simulink model "IEEE9_16b_0"  (R2020a)
settings: Solver=ode15s  StartTime=0.0  StopTime=5  MaxStep=1e-4  RelTol=1e-3
libraries: powerlib x23, sps_avr x3, simulink_extras x2, powerlib_meascontrol x2
settings Model: Creator=Pankaj  LastModifiedBy=ahmed
settings DataIOCC: ReturnWorkspaceOutputs=off
settings DebuggingCC: UnconnectedInputMsg=none  UnconnectedOutputMsg=none  UnconnectedLineMsg=none  ArithmeticOperatorsInVariantConditions=warning
settings SFSimCC: SimUseLocalCustomCode=off  CustomCodeUndefinedFunction=UseInterfaceOnly
settings RTWCC: RTWUseLocalCustomCode=off
settings CodeAppCC: StateflowObjectComments=on
settings SimscapeCC: SimscapeNormalizeSystem=off

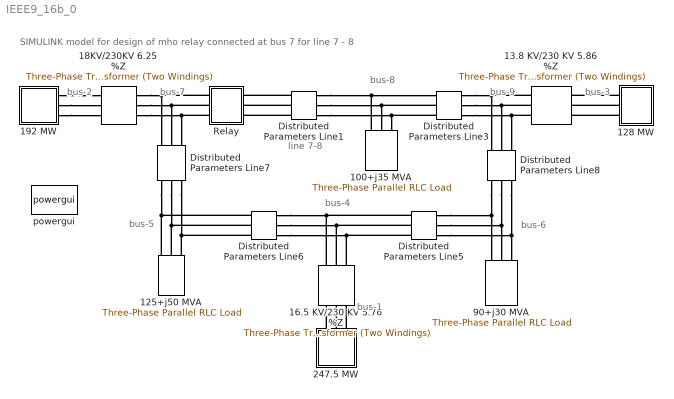
== system IEEE9_16b_0 ==
  note: SIMULINK model for design of mho relay connected at bus 7 for line 7 - 8
  note: bus-2
  note: bus-7
  note: bus-8
  note: bus-9
  note: bus-1
  note: bus-3
  note: bus-4
  note: bus-6
  note: bus-5
  note: line 7-8
  100+j35 MVA : powerlib/Elements/Three-Phase Parallel RLC Load  LConnTagsString=A|B|C  Configuration=Y (grounded)  NominalVoltage=(230000)*0.993698  Vabc=[1e3 1e3 1e3]  Vabcp=[1e3 1e3 1e3]  NominalFrequency=60  UnbalancedPower=off  ActivePower=100e6  InductivePower=35e6  CapacitivePower=0  Pabc=[10e3 9e3 11e3]  QLabc=[100 90 110]  QCabc=[100 90 110]  Pabcp=[10e3 9e3 11e3]  QLabcp=[100 90 110]  QCabcp=[100 90 110]  Measurements=None  LoadType=constant PQ
  125+j50 MVA : powerlib/Elements/Three-Phase Parallel RLC Load  LConnTagsString=A|B|C  Configuration=Y (grounded)  NominalVoltage=(223027)*1  Vabc=[1e3 1e3 1e3]  Vabcp=[1e3 1e3 1e3]  NominalFrequency=60  UnbalancedPower=off  ActivePower=125e6  InductivePower=50e6  CapacitivePower=0  Pabc=[10e3 9e3 11e3]  QLabc=[100 90 110]  QCabc=[100 90 110]  Pabcp=[10e3 9e3 11e3]  QLabcp=[100 90 110]  QCabcp=[100 90 110]  Measurements=None  LoadType=constant PQ
  128 MW : Subsystem
  13.8 KV/230 KV 5.86 %Z : powerlib/Elements/Three-Phase Transformer (Two Windings)  Winding1Connection=Yg  Winding2Connection=Yg  CoreType=Three single-phase transformers  SetSaturation=off  Hysteresis=off  DataFile='hysteresis'  SetInitialFlux=off  Measurements=None  UNITS=pu  NominalPower=[ 100e6 , 60 ]  Winding1=[13.8e3 , 1e-6 , 0 ]  Winding2=[ 230e3 , 1e-6, 0.0586 ]  Rm=500  Lm=500  L0=0.5  Saturation=[ 0,0 ; 0.0024,1.2 ; 1.0,1.52 ]  InitialFluxes=[ 0.8 , -0.8 , 0.7 ]  BreakLoop=off  DiscreteSolver=Trapezoidal iterative  DataType=off  TransfoNumber=1
  "16.5 KV/230 KV 5.76 %Z     " : powerlib/Elements/Three-Phase Transformer (Two Windings)  Winding1Connection=Yg  Winding2Connection=Yg  CoreType=Three single-phase transformers  SetSaturation=off  Hysteresis=off  DataFile='hysteresis'  SetInitialFlux=off  Measurements=None  UNITS=pu  NominalPower=[ 100e6 , 60 ]  Winding1=[16.5e3 , 1e-6, 0 ]  Winding2=[ 230e3 ,1e-6, 0.0576 ]  Rm=500  Lm=500  L0=0.5  Saturation=[ 0,0 ; 0.0024,1.2 ; 1.0,1.52 ]  InitialFluxes=[ 0.8 , -0.8 , 0.7 ]  BreakLoop=off  DiscreteSolver=Trapezoidal iterative  DataType=off  TransfoNumber=1
  18KV/230KV 6.25 %Z : powerlib/Elements/Three-Phase Transformer (Two Windings)  Winding1Connection=Yg  Winding2Connection=Yg  CoreType=Three single-phase transformers  SetSaturation=off  Hysteresis=off  DataFile='hysteresis'  SetInitialFlux=off  Measurements=None  UNITS=pu  NominalPower=[ 100e6 , 60 ]  Winding1=[ 18e3 , 1e-6 , 0]  Winding2=[ 230e3 , 1e-6, 0.0625 ]  Rm=500  Lm=500  L0=0.5  Saturation=[ 0,0 ; 0.0024,1.2 ; 1.0,1.52 ]  InitialFluxes=[ 0.8 , -0.8 , 0.7 ]  BreakLoop=off  DiscreteSolver=Trapezoidal iterative  DataType=off  TransfoNumber=1
  192 MW : Subsystem
  247.5 MW : Subsystem
  90+j30 MVA : powerlib/Elements/Three-Phase Parallel RLC Load  LConnTagsString=A|B|C  Configuration=Y (grounded)  NominalVoltage=(226177)*0.999999  Vabc=[1e3 1e3 1e3]  Vabcp=[1e3 1e3 1e3]  NominalFrequency=60  UnbalancedPower=off  ActivePower=90e6  InductivePower=30e6  CapacitivePower=0  Pabc=[10e3 9e3 11e3]  QLabc=[100 90 110]  QCabc=[100 90 110]  Pabcp=[10e3 9e3 11e3]  QLabcp=[100 90 110]  QCabcp=[100 90 110]  Measurements=None  LoadType=constant PQ
  Distributed Parameters Line1 : powerlib/Elements/Distributed Parameters Line  Phases=3  Frequency=60  Resistance=[0.044965 0.11241]  Inductance="[1.01e-3  2.02e-3]"  Capacitance=[12.74e-9 7.751e-9]  Length=100  x1=[-0.0004 1.93656449270455e-06 23508.2160177902 -52538.75935175;-0.00035 1.67378461087068e-06 24494.3184666325 -52086.3350065214;-0.0003 1.4104100413345e-06 25471.7182007562 -51615.4046344802;-0.00025 1.14653435982647e-06 26440.0679546897 -51126.1355549453;-0.0002 8.82251320119748e-07 27399.0236783764 -50618.7016028908;-0.00015 6.17654820719931e-07 28348.2446594139 -50093.2830671837;-0.0001 3.52838871503349e-07 29287.3936441074 -49550.0666265279;-5e-05 8.78975603158065e-08 30216.1369572946 -48989.2452831382]  x2=[-0.0004 4.18624145948892e-06 28259.244689254 -52398.8670670216;-0.00035 3.9633430905482e-06 29241.8663646278 -51856.9185470287;-0.0003 3.73903656467934e-06 30214.0985441207 -51296.5455107989;-0.00025 3.51340157692291e-06 31175.595798269 -50717.9470562037;-0.0002 3.28651829431568e-06 32126.0165116764 -50121.3287565189;-0.00015 3.05846732740762e-06 33065.023004389 -49506.9025873855;-0.0001 2.82932970162139e-06 33992.2816518711 -48874.8868514958;-5e-05 2.59918682846436e-06 34907.4630035407 -48225.5061010312]  x3=[-0.0004 -1.73044531826081e-08 87.9731080176391 -312.019576771818;-0.00035 -1.71851910893741e-08 93.8385916181453 -310.305999768085;-0.0003 -1.70598231795753e-08 99.6707348138731 -308.482172520194;-0.00025 -1.69283939958332e-08 105.467465472116 -306.54874302528;-0.0002 -1.67909502343109e-08 111.226724042071 -304.506398221637;-0.00015 -1.66475407281225e-08 116.946464286594 -302.355863744649;-0.0001 -1.64982164299825e-08 122.624654009211 -300.097903668976;-5e-05 -1.63430303941032e-08 128.259275776149 -297.733320237081]  x4=[-0.0004 3.28235405138543e-08 68.6553647797155 -68.5872480221798;-0.00035 3.17845507984995e-08 69.935937439127 -67.2810236786274;-0.0003 3.07342681835919e-08 71.1916621929746 -65.9508947077285;-0.00025 2.96730658295436e-08 72.4220928882326 -64.5973336979729;-0.0002 2.86013207764978e-08 73.6267923587337 -63.2208215631423;-0.00015 2.75194138103686e-08 74.8053325804924 -61.8218473714436;-0.0001 2.64277293275496e-08 75.9572948237797 -60.400908171746;-5e-05 2.53266551983393e-08 77.0822698018957 -58.9585088169809]  x5=0.000395689524753941  V1=ones(3,3)  V2=ones(3,3)  I1=ones(3,3)  I2=ones(3,3)  nHarmo=1  Measurements=None
  Distributed Parameters Line3 : powerlib/Elements/Distributed Parameters Line  Phases=3  Frequency=60  Resistance=[ 0.062951 0.15737]  Inductance="[ 1.414e-3  3.53e-3]"  Capacitance=[12.74e-9 7.751e-9]  Length=100  x1=[-0.00055 -3.66870332071984e-11 0 0;-0.0005 -3.60227656771721e-11 0 0;-0.00045 -3.53456994300274e-11 0 0;-0.0004 -3.46560750241779e-11 0 0;-0.00035 -3.39541374798913e-11 0 0;-0.0003 -3.32401361922348e-11 0 0;-0.00025 -3.25143248424659e-11 0 0;-0.0002 -3.17769613079014e-11 0 0;-0.00015 -3.10283075702939e-11 0 0;-0.0001 -3.02686296227516e-11 0 0;-5e-05 -2.9498197375232e-11 0 0]  x2=[-0.00055 6.0309326536538e-11 0 0;-0.0005 6.04326397123915e-11 0 0;-0.00045 6.05344814591124e-11 26135.3734716676 3233.45213495311;-0.0004 6.06148155928129e-11 26069.7846141014 3725.4882649243;-0.00035 6.0673613571158e-11 25994.9332861961 4216.20074665431;-0.0003 6.07108545035057e-11 25910.8460822721 4705.41523233496;-0.00025 6.07265251583303e-11 25817.5528781127 5192.95790638897;-0.0002 6.07206199679226e-11 25715.0868203491 5678.65554722571;-0.00015 6.06931410303687e-11 25603.4843146836 6162.33558878611;-0.0001 6.06440981088042e-11 25482.785012955 6643.82618185451;-5e-05 6.05735086279458e-11 25353.0317990507 7122.95625511585]  x3=[-0.00055 1.99765696866532e-13 0 0;-0.0005 2.12696705234761e-13 0 0;-0.00045 2.255521434764e-13 116.024829696429 -474.092172875078;-0.0004 2.38327444115455e-13 124.940123526668 -471.821073684818;-0.00035 2.5101806814844e-13 133.811026725934 -469.38233871371;-0.0003 2.63619506657064e-13 142.634387504562 -466.776834432677;-0.00025 2.76127282410229e-13 151.407070964479 -464.005486564982;-0.0002 2.88536951454765e-13 160.125960213026 -461.069279757328;-0.00015 3.00844104694353e-13 168.787957470368 -457.969257230012;-0.0001 3.13044369456047e-13 177.389985170124 -454.706520406277;-5e-05 3.25133411043871e-13 185.928987052813 -451.28222852098]  x4=[-0.00055 -2.34485159346315e-13 0 0;-0.0005 -2.46871311009831e-13 0 0;-0.00045 -2.59169750472053e-13 -37.9101805249176 477.43059089476;-0.0004 -2.71376108155999e-13 -46.9022764073901 476.631236412791;-0.00035 -2.83486047200907e-13 -55.8777081343857 475.662537122061;-0.0003 -2.95495265003096e-13 -64.8332867777495 474.524837196814;-0.00025 -3.07399494744665e-13 -73.7658304630324 473.218540856417;-0.0002 -3.19194506909471e-13 -82.6721654999966 471.74411222174;-0.00015 -3.30876110785854e-13 -91.5491275102119 470.102075150256;-0.0001 -3.42440155955581e-13 -100.393562551345 468.293013049917;-5e-05 -3.53882533768465e-13 -109.202328237739 466.317568671875]  x5=0.000523077718890797  V1=ones(3,3)  V2=ones(3,3)  I1=ones(3,3)  I2=ones(3,3)  nHarmo=1  Measurements=None
  Distributed Parameters Line5 : powerlib/Elements/Distributed Parameters Line  Phases=3  Frequency=60  Resistance=[ 0.08993 0.224825]  Inductance="[ 1.29e-3  3.22e-3]"  Capacitance=[12.74e-9 7.751e-9]  Length=100  x1=[-0.0005 9.3934579093273e-11 48708.3011698947 -2975.91430508471;-0.00045 9.415092660108e-11 48755.7392345492 -2057.30749504863;-0.0004 9.43338227329765e-11 48785.85461721 -1137.96973345567;-0.00035 9.44832025068375e-11 48798.6366180249 -218.227656634997;-0.0003 9.45990128487408e-11 48794.0806956099 701.591955432963;-0.00025 9.46812126118233e-11 48772.1884686624 1621.16229521987;-0.0002 9.47297725909006e-11 48732.9677153866 2540.15664376264;-0.00015 9.47446755328433e-11 48676.4323707293 3458.24848674514;-0.0001 9.47259161427072e-11 48602.6025214293 4375.11163050716;-5e-05 9.46735010856142e-11 48511.5043988804 5290.42031793947]  x2=[-0.0005 5.85167207852729e-11 40015.4206134486 -3326.82844604819;-0.00045 5.87167241813035e-11 40071.0170008075 -2572.00768036554;-0.0004 5.8895865804819e-11 40112.3763466289 -1816.27309260098;-0.00035 5.90540820076537e-11 40139.4839561341 -1059.89319165501;-0.0003 5.9191316576344e-11 40152.3301981187 -303.136715704854;-0.00025 5.93075207521012e-11 40150.9105083739 453.727463276971;-0.0002 5.9402653248135e-11 40135.2253913087 1210.43043505157;-0.00015 5.94766802643224e-11 40105.2804197707 1966.7033466562;-0.0001 5.95295754992172e-11 40061.0862330655 2722.27749792646;-5e-05 5.95613201593942e-11 40002.6585331773 3476.88443696415]  x3=[-0.0005 8.69475041814123e-14 110.762184106389 149.128598468394;-0.00045 8.25552456581707e-14 107.931686449283 151.189801864665;-0.0004 7.81336556492433e-14 105.062841177911 153.197288244241;-0.00035 7.36843051245063e-14 102.156667579338 155.150344356771;-0.0003 6.92087749170151e-14 99.2141982032043 157.048276290718;-0.00025 6.47086551613417e-14 96.2364784948694 158.890409719903;-0.0002 6.01855447286073e-14 93.2245664239666 160.676090143089;-0.00015 5.56410506584114e-14 90.1795321085132 162.404683116526;-0.0001 5.1076787587858e-14 87.1024574347021 164.075574479361;-5e-05 4.64943771778828e-14 83.9944356725131 165.688170571848]  x4=[-0.0005 1.05776183792212e-13 160.713797226438 -189.568367256825;-0.00045 1.09353327185716e-13 164.258290736407 -186.505475277131;-0.0004 1.1289161786277e-13 167.744424057812 -183.37631879014;-0.00035 1.16389798685544e-13 171.170958584084 -180.18200957025;-0.0003 1.19846626767049e-13 174.536676883822 -176.923682540318;-0.00025 1.23260873912727e-13 177.84038313334 -173.602495368422;-0.0002 1.26631327056826e-13 181.080903541539 -170.219628056551;-0.00015 1.29956788693391e-13 184.257086766948 -166.776282521352;-0.0001 1.33236077301738e-13 187.367804326791 -163.273682167098;-5e-05 1.36468027766239e-13 190.411950997929 -159.713071451017]  x5=0.000499582025297148  V1=ones(3,3)  V2=ones(3,3)  I1=ones(3,3)  I2=ones(3,3)  nHarmo=1  Measurements=None
  Distributed Parameters Line6 : powerlib/Elements/Distributed Parameters Line  Phases=3  Frequency=60  Resistance=[ 0.0529 0.13225]  Inductance="[ 1.192e-3  2.38e-3]"  Capacitance=[12.74e-9 7.751e-9]  Length=100  x1=[-0.00045 -7.51799567936038e-11 0 0;-0.0004 -7.27831003605691e-11 30956.489181022 -3720.43098085035;-0.00035 -7.03603844385416e-11 31021.1138221492 -3136.28684704199;-0.0003 -6.79126698069524e-11 31074.716809246 -2551.02840545068;-0.00025 -6.54408261271549e-11 31117.2790974264 -1964.86359561394;-0.0002 -6.29457316334387e-11 31148.7855645122 -1378.0006790976;-0.00015 -6.04282728209967e-11 31169.2250164054 -790.648165501498;-0.0001 -5.78893441309577e-11 31178.5901910663 -203.014738376955;-5e-05 -5.53298476325959e-11 31176.8777610929 384.690818917456]  x2=[-0.00045 9.53544713850958e-11 0 0;-0.0004 9.55062550114663e-11 48785.85461721 -1137.96973345567;-0.00035 9.56241057201955e-11 48798.6366180249 -218.227656634997;-0.0003 9.57079816394878e-11 48794.0806956099 701.591955432965;-0.00025 9.57578529686284e-11 48772.1884686624 1621.16229521987;-0.0002 9.57737019885716e-11 48732.9677153866 2540.15664376265;-0.00015 9.57555230682361e-11 48676.4323707293 3458.24848674515;-0.0001 9.57033226665056e-11 48602.6025214293 4375.11163050716;-5e-05 9.56171193299344e-11 48511.5043988804 5290.42031793947]  x3=[-0.00045 1.40009495986436e-12 0 0;-0.0004 1.43390486700962e-12 201.042404247823 -402.175025567488;-0.00035 1.46720531458334e-12 208.587038318217 -398.314235079061;-0.0003 1.49998447109506e-12 216.057562407109 -394.311925439531;-0.00025 1.53223069026655e-12 223.451322272861 -390.169518650454;-0.0002 1.56393251516969e-12 230.765690947799 -385.888486489239;-0.00015 1.59507868229704e-12 237.998069671561 -381.470349986228;-0.0001 1.62565812556372e-12 245.145888814425 -376.916678884283;-5e-05 1.65565998023915e-12 252.206608790285 -372.229091081064]  x4=[-0.00045 -1.35484476552596e-12 0 0;-0.0004 -1.38423587214648e-12 55.1323292586217 367.477676628513;-0.00035 -1.41313516635283e-12 48.1961742895283 368.451558015141;-0.0003 -1.44153238036338e-12 41.2428954492016 369.294530317632;-0.00025 -1.46941742478322e-12 34.2749632045046 370.006294031941;-0.0002 -1.49678039218884e-12 27.2948532285854 370.586596271809;-0.00015 -1.52361156064821e-12 20.3050455212818 371.035230858613;-0.0001 -1.54990139717493e-12 13.3080235279893 371.352038394622;-5e-05 -1.57564056111528e-12 6.30627325730502 371.536906319625]  x5=0.000429504132692574  V1=ones(3,3)  V2=ones(3,3)  I1=ones(3,3)  I2=ones(3,3)  nHarmo=1  Measurements=None
  Distributed Parameters Line7 : powerlib/Elements/Distributed Parameters Line  Phases=3  Frequency=60  Resistance=[ 0.16928 0.4232]  Inductance="[ 2.259e-3  5.64e-3]"  Capacitance=[12.74e-9 7.751e-9]  Length=100  x1=[-0.0007 -8.67468793349911e-11 30338.8453774411 -7190.30986678695;-0.00065 -8.4491899948746e-11 30468.9813561391 -6617.19098742957;-0.0006 -8.22069009927673e-11 30588.2918508428 -6041.72105162289;-0.00055 -7.98926943163037e-11 30696.7344711017 -5464.10452109494;-0.0005 -7.7550102145968e-11 30794.2706877692 -4884.54662024862;-0.00045 -7.51799567936038e-11 30880.8658466918 -4303.25326324648;-0.0004 -7.27831003605691e-11 30956.489181022 -3720.43098085034;-0.00035 -7.03603844385416e-11 31021.1138221492 -3136.28684704199;-0.0003 -6.79126698069524e-11 31074.716809246 -2551.02840545068;-0.00025 -6.54408261271549e-11 31117.2790974264 -1964.86359561394;-0.0002 -6.29457316334387e-11 31148.7855645122 -1378.0006790976;-0.00015 -6.04282728209967e-11 31169.2250164054 -790.648165501498;-0.0001 -5.78893441309577e-11 31178.5901910663 -203.014738376955;-5e-05 -5.53298476325959e-11 31176.8777610929 384.690818917456]  x2=[-0.0007 3.36738686208368e-10 0 0;-0.00065 3.33752277633264e-10 0 0;-0.0006 3.30647288463118e-10 0 0;-0.00055 3.27424821885796e-10 0 0;-0.0005 3.24086022828331e-10 0 0;-0.00045 3.20632077550129e-10 0 0;-0.0004 3.17064213221501e-10 0 0;-0.00035 3.13383697487653e-10 0 0;-0.0003 3.09591838018302e-10 0 0;-0.00025 3.05689982043061e-10 0 0;-0.0002 3.01679515872779e-10 0 0;-0.00015 2.9756186440699e-10 0 0;-0.0001 2.93338490627653e-10 0 0;-5e-05 2.89010895079362e-10 0 0]  x3=[-0.0007 1.45033859622586e-12 81.7335914900186 330.37653858012;-0.00065 1.48313751388857e-12 75.4920072838225 331.858404494915;-0.0006 1.51540947985473e-12 69.2236011269026 333.222362698776;-0.00055 1.5471430280485e-12 62.9306001541187 334.467928583847;-0.0005 1.57832688369131e-12 56.6152402387514 335.594659606501;-0.00045 1.60894996730773e-12 50.2797651981075 336.60215544457;-0.0004 1.63900139866197e-12 43.9264259963018 337.490058139581;-0.00035 1.66847050062357e-12 37.5574799445004 338.258052223934;-0.0003 1.69734680296091e-12 31.1751898989091 338.905864832987;-0.00025 1.72562004606128e-12 24.781823456791 339.433265802005;-0.0002 1.75328018457602e-12 18.3796521508004 339.840067747935;-0.00015 1.78031739098964e-12 11.9709506419174 340.126126135983;-0.0001 1.80672205911143e-12 5.55799591127248 340.291339330966;-5e-05 1.83248480748854e-12 -0.85693354885468 340.335648633421]  x4=[-0.0007 -1.18899619904894e-12 -13.5268241568473 -354.109143670938;-0.00065 -1.22204150654777e-12 -6.85003572889313 -354.301198747101;-0.0006 -1.25465262851822e-12 -0.170813515861694 -354.367372294396;-0.00055 -1.28681797838393e-12 6.50846938639857 -354.307640801677;-0.0005 -1.31852612794926e-12 13.1854398604767 -354.122025491259;-0.00045 -1.34976581145964e-12 19.8577256105564 -353.810592311378;-0.0004 -1.38052592960428e-12 26.5229560052816 -353.373451912759;-0.00035 -1.41079555345967e-12 33.1787629200303 -352.810759609305;-0.0003 -1.44056392837259e-12 39.8227815782981 -352.122715322912;-0.00025 -1.46982047778117e-12 46.4526513918921 -351.309563512439;-0.0002 -1.49855480697272e-12 53.0660167996362 -350.371593086851;-0.00015 -1.52675670677689e-12 59.6605281042916 -349.309137302576;-0.0001 -1.55441615719298e-12 66.2338423073921 -348.122573645093;-5e-05 -1.58152333094996e-12 72.7836239417011 -346.812323694822]  x5=0.000661178039562719  V1=ones(3,3)  V2=ones(3,3)  I1=ones(3,3)  I2=ones(3,3)  nHarmo=1  Measurements=None
  Distributed Parameters Line8 : powerlib/Elements/Distributed Parameters Line  Phases=3  Frequency=60  Resistance=[ 0.20631 0.5157]  Inductance="[ 2.38e-3  6.09e-3]"  Capacitance=[12.74e-9 7.751e-9]  Length=100  x1=[-0.0007 5.79486260567101e-11 39651.1354266259 -6331.61647352943;-0.00065 5.82334499707458e-11 39763.4319813253 -5583.12816330729;-0.0006 5.84975838172923e-11 39861.6007779799 -4832.65619423344;-0.00055 5.87409337508517e-11 39945.6069376839 -4080.46720542505;-0.0005 5.89634133103513e-11 40015.4206134486 -3326.82844604819;-0.00045 5.9164943449863e-11 40071.0170008075 -2572.00768036554;-0.0004 5.93454525666878e-11 40112.3763466289 -1816.27309260098;-0.00035 5.95048765267961e-11 40139.4839561341 -1059.89319165501;-0.0003 5.96431586876138e-11 40152.3301981187 -303.136715704854;-0.00025 5.97602499181478e-11 40150.9105083739 453.727463276971;-0.0002 5.98561086164414e-11 40135.2253913087 1210.43043505157;-0.00015 5.99307007243554e-11 40105.2804197707 1966.7033466562;-0.0001 5.99839997396692e-11 40061.0862330655 2722.27749792646;-5e-05 6.00159867254964e-11 40002.6585331773 3476.88443696415]  x2=[-0.0007 5.98110346074028e-11 26323.6806978282 759.548372622182;-0.00065 5.99984687608999e-11 26304.6876597042 1255.5732434814;-0.0006 6.0164585744136e-11 26276.3486913077 1751.15201514576;-0.00055 6.0309326536538e-11 26238.6738613391 2246.10861083746;-0.0005 6.04326397123915e-11 26191.676555486 2740.26717483485;-0.00045 6.05344814591124e-11 26135.3734716676 3233.45213495311;-0.0004 6.06148155928129e-11 26069.7846141014 3725.4882649243;-0.00035 6.0673613571158e-11 25994.9332861961 4216.20074665431;-0.0003 6.07108545035057e-11 25910.8460822721 4705.41523233496;-0.00025 6.07265251583303e-11 25817.5528781127 5192.95790638897;-0.0002 6.07206199679226e-11 25715.0868203491 5678.65554722571;-0.00015 6.06931410303687e-11 25603.4843146836 6162.33558878611;-0.0001 6.06440981088042e-11 25482.785012955 6643.82618185451;-5e-05 6.05735086279458e-11 25353.0317990507 7122.95625511585]  x3=[-0.0007 7.20284598390996e-14 129.259203687359 132.178534568252;-0.00065 7.19782344672079e-14 126.744901415185 134.59138830833;-0.0006 7.19024355713429e-14 124.18556728305 136.956422369015;-0.00055 7.18010900824914e-14 121.582110610182 139.272796464966;-0.0005 7.16742340082229e-14 118.935456392343 141.539687599496;-0.00045 7.15219124198966e-14 116.246544973173 143.756290356981;-0.0004 7.13441794366475e-14 113.516331710095 145.921817189014;-0.00035 7.11410982061583e-14 110.745786634882 148.035498694224;-0.0003 7.09127408822232e-14 107.935894109007 150.096583891637;-0.00025 7.0659188599112e-14 105.087652473904 152.104340487495;-0.0002 7.03805314427437e-14 102.202073696265 154.058055135441;-0.00015 7.00768684186789e-14 99.2801830084886 155.957033689963;-0.0001 6.97483074169443e-14 96.3230185444237 157.800601453023;-5e-05 6.93949651736992e-14 93.3316309705233 159.588103413773]  x4=[-0.0007 5.42022948298432e-14 16.694766903928 -160.141714708115;-0.00065 5.44013295730297e-14 19.7102006457955 -159.798594306567;-0.0006 5.45810357828573e-14 22.718631447226 -159.398698225361;-0.00055 5.47413496105654e-14 25.7189904270807 -158.942168545671;-0.0005 5.48822140974141e-14 28.7102115721006 -158.429167470319;-0.00045 5.50035791949222e-14 31.6912321156561 -157.859877266144;-0.0004 5.51054017826484e-14 34.6609929153424 -157.234500199245;-0.00035 5.51876456835121e-14 37.6184388292883 -156.553258463116;-0.0003 5.52502816766469e-14 40.5625190910428 -155.816394099701;-0.00025 5.52932875077828e-14 43.4921876829075 -155.024168913401;-0.0002 5.53166478971526e-14 46.4064037075816 -154.176864378052;-0.00015 5.53203545449213e-14 49.304131757988 -153.274781536921;-0.0001 5.53044061341346e-14 52.1843422851482 -152.318240895746;-5e-05 5.5268808331187e-14 55.0460119639764 -151.307582308862]  x5=0.000687048688231045  V1=ones(3,3)  V2=ones(3,3)  I1=ones(3,3)  I2=ones(3,3)  nHarmo=1  Measurements=None
  Relay : Subsystem
  powergui : powerlib/powergui  Priority=1  SimulationMode=Discrete  SampleTime=50e-6  frequency=60  Iterations=50  frequencyindice=60  Pbase=100e6  ErrMax=0.0001  UnitsV=kV  UnitsW=MW  buscounter=0  FunctionMessages=off  echomessages=off  EnableUseOfTLC=off  CurrentSourceSwitches=off  DisableSnubberDevices=off  DisableRonSwitches=off  DisableVfSwitches=off  DisplayEquations=off  AutomaticDiscreteSolvers=off  SolverType=Tustin/Backward Euler (TBE)  Interpol=off  ExternalGateDelay=off  methode=off  Ts=100  x0status=blocks  SPID=on  SwTol=0  HookPort=off  NonlinearTolerance=1e-4  nMaxIteration=100  ContinueOnMaxIteration=off  RestoreLinks=warning  ResistiveCurrentMeasurement=off  Frange=[0:2:500]  Ylog=off  Xlog=on  ShowGrid=off  save=off  variable=ZData  structure=0  ZoomFFT=off  StartTime=0.0  cycles=1  DisplayStyle=1  fundamental=60  FreqAxis=off  MaxFrequency=1000  frequencyindicesteady=1  RmsSteady=1  display=off
  connections:
  100+j35 MVA/LConn1 -- Distributed Parameters Line3/LConn1 -- Distributed Parameters Line1/RConn1
  Distributed Parameters Line3/LConn2 -- Distributed Parameters Line1/RConn2 -- 100+j35 MVA/LConn2
  Distributed Parameters Line5/RConn1 -- Distributed Parameters Line8/LConn1 -- 90+j30 MVA/LConn1
  Distributed Parameters Line5/RConn3 -- Distributed Parameters Line8/LConn3 -- 90+j30 MVA/LConn3
  Distributed Parameters Line6/LConn1 -- Distributed Parameters Line7/LConn1 -- 125+j50 MVA/LConn1
  Distributed Parameters Line6/LConn2 -- Distributed Parameters Line7/LConn2 -- 125+j50 MVA/LConn2
  Distributed Parameters Line6/LConn3 -- Distributed Parameters Line7/LConn3 -- 125+j50 MVA/LConn3
  Distributed Parameters Line3/RConn1 -- 13.8 KV/230 KV 5.86 %Z/RConn1 -- Distributed Parameters Line8/RConn1
  Distributed Parameters Line3/RConn2 -- 13.8 KV/230 KV 5.86 %Z/RConn2 -- Distributed Parameters Line8/RConn2
  Distributed Parameters Line3/RConn3 -- 13.8 KV/230 KV 5.86 %Z/RConn3 -- Distributed Parameters Line8/RConn3
  18KV/230KV 6.25 %Z/RConn1 -- Distributed Parameters Line7/RConn1 -- Relay/LConn1
  Distributed Parameters Line5/RConn2 -- Distributed Parameters Line8/LConn2 -- 90+j30 MVA/LConn2
  Distributed Parameters Line6/RConn1 -- "16.5 KV/230 KV 5.76 %Z     "/RConn1 -- Distributed Parameters Line5/LConn1
  Distributed Parameters Line6/RConn2 -- "16.5 KV/230 KV 5.76 %Z     "/RConn2 -- Distributed Parameters Line5/LConn2
  Distributed Parameters Line6/RConn3 -- "16.5 KV/230 KV 5.76 %Z     "/RConn3 -- Distributed Parameters Line5/LConn3
  247.5 MW/RConn1 -- "16.5 KV/230 KV 5.76 %Z     "/LConn1
  247.5 MW/RConn2 -- "16.5 KV/230 KV 5.76 %Z     "/LConn2
  247.5 MW/RConn3 -- "16.5 KV/230 KV 5.76 %Z     "/LConn3
  128 MW/RConn1 -- 13.8 KV/230 KV 5.86 %Z/LConn1
  128 MW/RConn2 -- 13.8 KV/230 KV 5.86 %Z/LConn2
  128 MW/RConn3 -- 13.8 KV/230 KV 5.86 %Z/LConn3
  192 MW/RConn1 -- 18KV/230KV 6.25 %Z/LConn1
  192 MW/RConn2 -- 18KV/230KV 6.25 %Z/LConn2
  192 MW/RConn3 -- 18KV/230KV 6.25 %Z/LConn3
  18KV/230KV 6.25 %Z/RConn3 -- Distributed Parameters Line7/RConn3 -- Relay/LConn3
  Distributed Parameters Line3/LConn3 -- Distributed Parameters Line1/RConn3 -- 100+j35 MVA/LConn3
  18KV/230KV 6.25 %Z/RConn2 -- Relay/LConn2 -- Distributed Parameters Line7/RConn2
  Distributed Parameters Line1/LConn1 -- Relay/RConn1
  Distributed Parameters Line1/LConn2 -- Relay/RConn2
  Distributed Parameters Line1/LConn3 -- Relay/RConn3

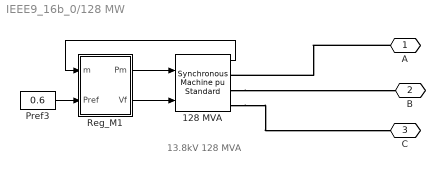
== system IEEE9_16b_0/128 MW ==
  note: 13.8kV 128 MVA
  128 MVA : powerlib/Machines/Synchronous Machine pu Standard  PresetModel=No  MechanicalLoad=Mechanical power Pm  ShowDetailedParameters=on  RotorType=Salient-pole  Units=per unit standard parameters  MeasurementBus=off  NominalParameters="[128e6  13800   60 ]"  Reactances1=[ 31 32 33 34 35 36 37 ]  Reactances2=[ 1.305, 0.296, 0.252, 0.474, 0.243, 0.18 ]  dAxisTimeConstants=Short-circuit  qAxisTimeConstants=Open-circuit  TimeConstants1=[]  TimeConstants2=[]  TimeConstants3=[]  TimeConstants4=[]  TimeConstants5=[ 1.01, 0.053, 0.1 ]  TimeConstants6=[]  TimeConstants7=[]  TimeConstants8=[]  StatorResistance=2.8544e-3  Mechanical="[20 0  32]"  PolePairs=32  InitialConditions=[0 -74.5248 0.603223 0.603223 0.603223 5.08525 -114.915 125.085 1.10339]  SetSaturation=off  Saturation=[0.6404,0.7127,0.8441,0.9214,0.9956,1.082,1.19,1.316,1.457;0.7,0.7698,0.8872,0.9466,0.9969,1.046,1.1,1.151,1.201]  LoadFlowParameters=[1 500000000 0 0 0]  TsPowergui=0  TsBlock=-1  IterativeModel=Trapezoidal non iterative  IterativeDiscreteModel=Trapezoidal non iterative  BusType=PV  Pref=0.6*128e6  Qref=0  Qmin=-Inf  Qmax=Inf  PLF=0  QLF=0
      settings: AttributesFormatString=\n\n
  Pref3 : Constant  Value=0.6
  Reg_M1 : Subsystem
  A : PMIOPort  Side=Right
  B : PMIOPort  Port=2  Side=Right
  C : PMIOPort  Port=3  Side=Right
  wires:
  Reg_M1/1(Pm) -> 128 MVA/1
  Reg_M1/2(Vf) -> 128 MVA/2
  Pref3/1 -> Reg_M1/2(Pref)
  128 MVA/1 -> Reg_M1/1(m)
  connections:
  A/RConn1 -- 128 MVA/RConn1
  128 MVA/RConn2 -- B/RConn1
  128 MVA/RConn3 -- C/RConn1

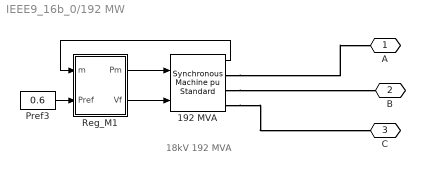
== system IEEE9_16b_0/192 MW ==
  note: 18kV 192 MVA
  192 MVA : powerlib/Machines/Synchronous Machine pu Standard  PresetModel=No  MechanicalLoad=Mechanical power Pm  ShowDetailedParameters=on  RotorType=Salient-pole  Units=per unit standard parameters  MeasurementBus=off  NominalParameters="[192e6  18000   60 ]"  Reactances1=[ 31 32 33 34 35 36 37 ]  Reactances2=[ 1.305, 0.296, 0.252, 0.474, 0.243, 0.18 ]  dAxisTimeConstants=Short-circuit  qAxisTimeConstants=Open-circuit  TimeConstants1=[]  TimeConstants2=[]  TimeConstants3=[]  TimeConstants4=[]  TimeConstants5=[ 1.01, 0.053, 0.1 ]  TimeConstants6=[]  TimeConstants7=[]  TimeConstants8=[]  StatorResistance=2.8544e-3  Mechanical="[20 0  32]"  PolePairs=32  InitialConditions=[0 -73.0594 0.600015 0.600015 0.600015 0.71576 -119.284 120.716 1.18255]  SetSaturation=off  Saturation=[0.6404,0.7127,0.8441,0.9214,0.9956,1.082,1.19,1.316,1.457;0.7,0.7698,0.8872,0.9466,0.9969,1.046,1.1,1.151,1.201]  LoadFlowParameters=[1 500000000 0 0 0]  TsPowergui=0  TsBlock=-1  IterativeModel=Trapezoidal non iterative  IterativeDiscreteModel=Trapezoidal non iterative  BusType=PV  Pref=0.6*192e6  Qref=0  Qmin=-Inf  Qmax=Inf  PLF=0  QLF=0
      settings: AttributesFormatString=\n\n
  Pref3 : Constant  Value=0.6
  Reg_M1 : Subsystem
  A : PMIOPort  Side=Right
  B : PMIOPort  Port=2  Side=Right
  C : PMIOPort  Port=3  Side=Right
  wires:
  Reg_M1/1(Pm) -> 192 MVA/1
  192 MVA/1 -> Reg_M1/1(m)
  Reg_M1/2(Vf) -> 192 MVA/2
  Pref3/1 -> Reg_M1/2(Pref)
  connections:
  192 MVA/RConn1 -- A/RConn1
  192 MVA/RConn3 -- C/RConn1
  192 MVA/RConn2 -- B/RConn1

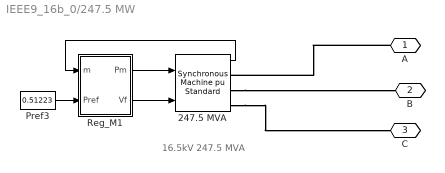
== system IEEE9_16b_0/247.5 MW ==
  note: 16.5kV 247.5 MVA
  247.5 MVA : powerlib/Machines/Synchronous Machine pu Standard  PresetModel=No  MechanicalLoad=Mechanical power Pm  ShowDetailedParameters=on  RotorType=Salient-pole  Units=per unit standard parameters  MeasurementBus=off  NominalParameters="[247.5e6  16500   60 ]"  Reactances1=[ 31 32 33 34 35 36 37 ]  Reactances2=[ 1.305, 0.296, 0.252, 0.474, 0.243, 0.18 ]  dAxisTimeConstants=Short-circuit  qAxisTimeConstants=Open-circuit  TimeConstants1=[]  TimeConstants2=[]  TimeConstants3=[]  TimeConstants4=[]  TimeConstants5=[ 1.01, 0.053, 0.1 ]  TimeConstants6=[]  TimeConstants7=[]  TimeConstants8=[]  StatorResistance=2.8544e-3  Mechanical=[20 0 32]  PolePairs=32  InitialConditions=[0 -76.6925 0.514814 0.514814 0.514814 -5.74321 -125.743 114.257 1.19383]  SetSaturation=off  Saturation=[0.6404,0.7127,0.8441,0.9214,0.9956,1.082,1.19,1.316,1.457;0.7,0.7698,0.8872,0.9466,0.9969,1.046,1.1,1.151,1.201]  LoadFlowParameters=[1 500000000 0 0 0]  TsPowergui=0  TsBlock=-1  IterativeModel=Trapezoidal non iterative  IterativeDiscreteModel=Trapezoidal non iterative  BusType=swing  Pref=5e+008  Qref=0  Qmin=-Inf  Qmax=Inf  PLF=0  QLF=0
      settings: AttributesFormatString=\n\n
  Pref3 : Constant  Value=0.51223
  Reg_M1 : Subsystem
  A : PMIOPort  Side=Right
  B : PMIOPort  Port=2  Side=Right
  C : PMIOPort  Port=3  Side=Right
  wires:
  Reg_M1/1(Pm) -> 247.5 MVA/1
  Reg_M1/2(Vf) -> 247.5 MVA/2
  Pref3/1 -> Reg_M1/2(Pref)
  247.5 MVA/1 -> Reg_M1/1(m)
  connections:
  A/RConn1 -- 247.5 MVA/RConn1
  247.5 MVA/RConn2 -- B/RConn1
  247.5 MVA/RConn3 -- C/RConn1

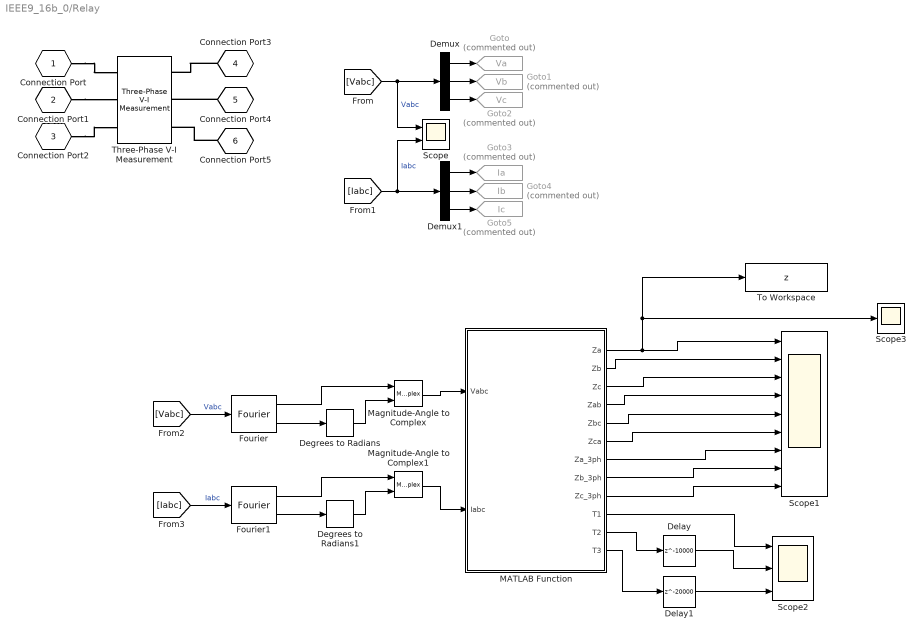
== system IEEE9_16b_0/Relay ==
  Degrees to Radians : simulink_extras/Transformations/Degrees to Radians
  Degrees to Radians1 : simulink_extras/Transformations/Degrees to Radians
  Delay : Delay  DelayLength=10000  SampleTime=50e-6
  Delay1 : Delay  DelayLength=20000  SampleTime=50e-6
  Demux : Demux  Outputs=3
  Demux1 : Demux  Outputs=3
  Fourier : powerlib_meascontrol/Measurements/Fourier  Freq=60  n=1  InInit=[0, 0]  Ts=0
  Fourier1 : powerlib_meascontrol/Measurements/Fourier  Freq=60  n=1  InInit=[0, 0]  Ts=0
  Goto : Goto  Commented=on  GotoTag=Va  TagVisibility=global
  Goto1 : Goto  Commented=on  GotoTag=Vb  TagVisibility=global
  Goto2 : Goto  Commented=on  GotoTag=Vc  TagVisibility=global
  Goto3 : Goto  Commented=on  GotoTag=Ia  TagVisibility=global
  Goto4 : Goto  Commented=on  GotoTag=Ib  TagVisibility=global
  Goto5 : Goto  Commented=on  GotoTag=Ic  TagVisibility=global
  MATLAB Function : MATLAB Function  TreatAsAtomicUnit=on
  Magnitude-Angle to Complex : MagnitudeAngleToComplex
  Magnitude-Angle to Complex1 : MagnitudeAngleToComplex
  Scope : Scope  NumInputPorts=2
  Scope1 : Scope  NumInputPorts=9
  Scope2 : Scope  NumInputPorts=3
  Scope3 : Scope
  Three-Phase V-I Measurement : powerlib/Measurements/Three-Phase V-I Measurement  VoltageMeasurement=phase-to-ground  SetLabelV=on  LabelV=Vabc  Vpu=off  VpuLL=off  CurrentMeasurement=yes  SetLabelI=on  LabelI=Iabc  Ipu=off  Pbase=100e6  Vbase=500e3  OutputType=Complex  PhasorSimulation=off  PSBequivalent=0
  To Workspace : ToWorkspace  VariableName=z  SampleTime=-1
  Connection Port : PMIOPort  Tag=PMCPort  Side=Left
  Connection Port1 : PMIOPort  Tag=PMCPort  Port=2  Side=Left
  Connection Port2 : PMIOPort  Tag=PMCPort  Port=3  Side=Left
  Connection Port3 : PMIOPort  Tag=PMCPort  Port=4  Side=Right
  Connection Port4 : PMIOPort  Tag=PMCPort  Port=5  Side=Right
  Connection Port5 : PMIOPort  Tag=PMCPort  Port=6  Side=Right
  wires:
  Demux1/3 -> Goto5/1
  Demux1/1 -> Goto3/1
  Demux/3 -> Goto2/1
  Demux/1 -> Goto/1
  Demux/2 -> Goto1/1
  [Iabc] -> Scope/2, Demux1/1  "Iabc"
  [Vabc] -> Scope/1, Demux/1  "Vabc"
  Demux1/2 -> Goto4/1
  MATLAB Function/1(Za) -> Scope3/1, To Workspace/1, Scope1/1
  MATLAB Function/2(Zb) -> Scope1/2
  MATLAB Function/3(Zc) -> Scope1/3
  MATLAB Function/4(Zab) -> Scope1/4
  MATLAB Function/5(Zbc) -> Scope1/5
  MATLAB Function/6(Zca) -> Scope1/6
  MATLAB Function/10(T1) -> Scope2/1
  Fourier/2 -> Degrees to Radians/1
  Degrees to Radians/1 -> Magnitude-Angle to Complex/2
  Fourier/1 -> Magnitude-Angle to Complex/1
  Magnitude-Angle to Complex/1 -> MATLAB Function/1(Vabc)
  [Vabc] -> Fourier/1  "Vabc"
  Fourier1/1 -> Magnitude-Angle to Complex1/1
  Degrees to Radians1/1 -> Magnitude-Angle to Complex1/2
  Fourier1/2 -> Degrees to Radians1/1
  [Iabc] -> Fourier1/1  "Iabc"
  Magnitude-Angle to Complex1/1 -> MATLAB Function/2(Iabc)
  MATLAB Function/11(T2) -> Delay/1
  MATLAB Function/12(T3) -> Delay1/1
  Delay/1 -> Scope2/2
  Delay1/1 -> Scope2/3
  MATLAB Function/7(Za_3ph) -> Scope1/7
  MATLAB Function/8(Zb_3ph) -> Scope1/8
  MATLAB Function/9(Zc_3ph) -> Scope1/9
  connections:
  Connection Port/RConn1 -- Three-Phase V-I Measurement/LConn1
  Connection Port1/RConn1 -- Three-Phase V-I Measurement/LConn2
  Connection Port2/RConn1 -- Three-Phase V-I Measurement/LConn3
  Connection Port3/RConn1 -- Three-Phase V-I Measurement/RConn1
  Connection Port4/RConn1 -- Three-Phase V-I Measurement/RConn2
  Connection Port5/RConn1 -- Three-Phase V-I Measurement/RConn3

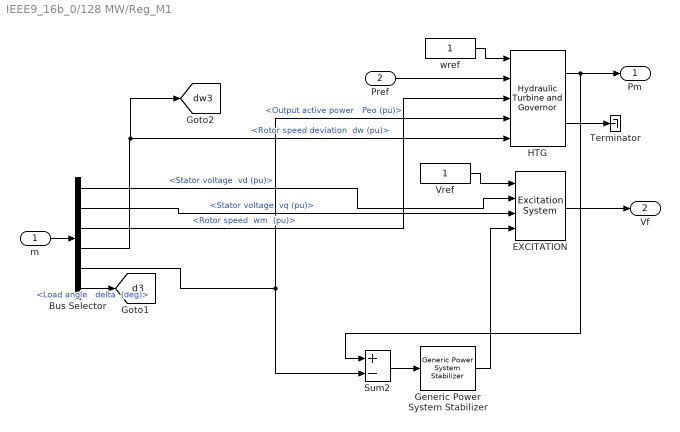
== system IEEE9_16b_0/128 MW/Reg_M1 ==
  m : Inport
  Pref : Inport  Port=2
  Bus Selector : BusSelector  OutputSignals="dq0 components.Stator voltage  vd (pu),dq0 components.Stator voltage  vq (pu),Mechanical.Rotor speed  wm  (pu),Mechanical.Rotor speed deviation  dw (pu),Output active power   Peo (pu),Load angle   delta  (deg)"
  EXCITATION : sps_avr/Excitation System  tr=20e-3  reg=[ 200, 0.001 ]  exc=[ 1, 0 ]  tgr=[ 0, 0 ]  damp=[ 0.001, 0.1 ]  sat=[ 0, 0 ]  lim="[ 0,  7, 0 ]"  v0=[1 1.1034]
      settings: SourceProductBaseCode=PS
  Generic Power System Stabilizer : powerlib/Machines/Generic Power System Stabilizer  Tsensor=15e-3  K=2.5  Twashout=1  Tleadlag1="[0.06  1]"  Tleadlag2="[0  0]"  VSlimits=[-0.15 0.15]  Vinit=0  Plot_On=off  MagdB_On=on  FreqRange=logspace(-2,2,500)
      settings: SourceProductBaseCode=PS
  HTG : powerlib/Machines/Hydraulic Turbine and Governor  sm="[ 10/3  0.07 ]"  gate="[  0.01  0.97518  -0.1  0.1 ]"  reg="[  0.05  1.163  0.105  0  0.01  ]"  hyd="[  0  2.67  ]"  dref=0  po=0.60104
      settings: SourceProductBaseCode=PS
  Sum2 : Sum  Inputs=+-  InputSameDT=on  SaturateOnIntegerOverflow=on  OutDataTypeStr=Inherit: Same as first input
  Terminator : Terminator
  Vref : Constant
  wref : Constant
  Pm : Outport  InitialOutput=0
  Vf : Outport  Port=2  InitialOutput=0
  tag scope: d3=global, dw3=global
  wires:
  HTG/2 -> Terminator/1
  Vref/1 -> EXCITATION/1
  m/1 -> Bus Selector/1
  Bus Selector/4 -> [dw3], HTG/5  "<Rotor speed deviation  dw (pu)>"
  Bus Selector/5 -> HTG/4, Sum2/2  "<Output active power   Peo (pu)>"
  Bus Selector/3 -> HTG/3  "<Rotor speed  wm  (pu)>"
  Pref/1 -> HTG/2
  wref/1 -> HTG/1
  HTG/1 -> Pm/1, Sum2/1
  Bus Selector/2 -> EXCITATION/3  "<Stator voltage  vq (pu)>"
  EXCITATION/1 -> Vf/1
  Bus Selector/1 -> EXCITATION/2  "<Stator voltage  vd (pu)>"
  Generic Power System Stabilizer/1 -> EXCITATION/4
  Sum2/1 -> Generic Power System Stabilizer/1
  Bus Selector/6 -> [d3]  "<Load angle   delta  (deg)>"

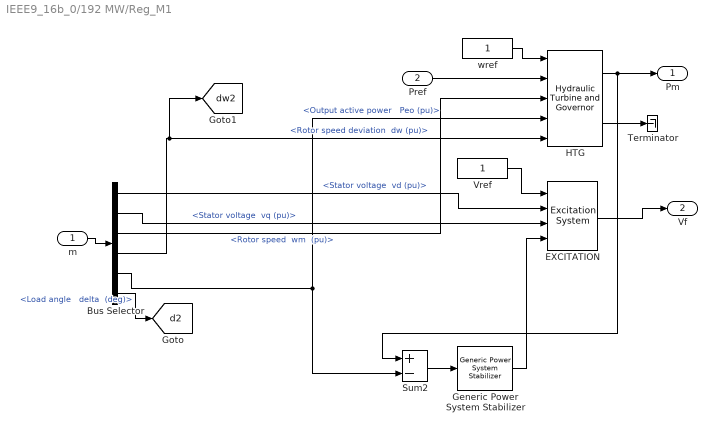
== system IEEE9_16b_0/192 MW/Reg_M1 ==
  m : Inport
  Pref : Inport  Port=2
  Bus Selector : BusSelector  OutputSignals="dq0 components.Stator voltage  vd (pu),dq0 components.Stator voltage  vq (pu),Mechanical.Rotor speed  wm  (pu),Mechanical.Rotor speed deviation  dw (pu),Output active power   Peo (pu),Load angle   delta  (deg)"
  EXCITATION : sps_avr/Excitation System  tr=20e-3  reg=[ 200, 0.001 ]  exc=[ 1, 0 ]  tgr=[ 0, 0 ]  damp=[ 0.001, 0.1 ]  sat=[ 0, 0 ]  lim="[ 0,  7, 0 ]"  v0=[1 1.1826]
      settings: SourceProductBaseCode=PS
  Generic Power System Stabilizer : powerlib/Machines/Generic Power System Stabilizer  Tsensor=15e-3  K=2.5  Twashout=1  Tleadlag1="[0.06  1]"  Tleadlag2="[0  0]"  VSlimits=[-0.15 0.15]  Vinit=0  Plot_On=off  MagdB_On=on  FreqRange=logspace(-2,2,500)
      settings: SourceProductBaseCode=PS
  HTG : powerlib/Machines/Hydraulic Turbine and Governor  sm="[ 10/3  0.07 ]"  gate="[  0.01  0.97518  -0.1  0.1 ]"  reg="[  0.05  1.163  0.105  0  0.01  ]"  hyd="[  0  2.67  ]"  dref=0  po=0.60103
      settings: SourceProductBaseCode=PS
  Sum2 : Sum  Inputs=+-  InputSameDT=on  SaturateOnIntegerOverflow=on  OutDataTypeStr=Inherit: Same as first input
  Terminator : Terminator
  Vref : Constant
  wref : Constant
  Pm : Outport  InitialOutput=0
  Vf : Outport  Port=2  InitialOutput=0
  tag scope: d2=global, dw2=global
  wires:
  HTG/2 -> Terminator/1
  Vref/1 -> EXCITATION/1
  m/1 -> Bus Selector/1
  Bus Selector/4 -> [dw2], HTG/5  "<Rotor speed deviation  dw (pu)>"
  Bus Selector/5 -> HTG/4, Sum2/2  "<Output active power   Peo (pu)>"
  Bus Selector/3 -> HTG/3  "<Rotor speed  wm  (pu)>"
  Pref/1 -> HTG/2
  wref/1 -> HTG/1
  HTG/1 -> Pm/1, Sum2/1
  Bus Selector/2 -> EXCITATION/3  "<Stator voltage  vq (pu)>"
  EXCITATION/1 -> Vf/1
  Bus Selector/1 -> EXCITATION/2  "<Stator voltage  vd (pu)>"
  Generic Power System Stabilizer/1 -> EXCITATION/4
  Sum2/1 -> Generic Power System Stabilizer/1
  Bus Selector/6 -> [d2]  "<Load angle   delta  (deg)>"

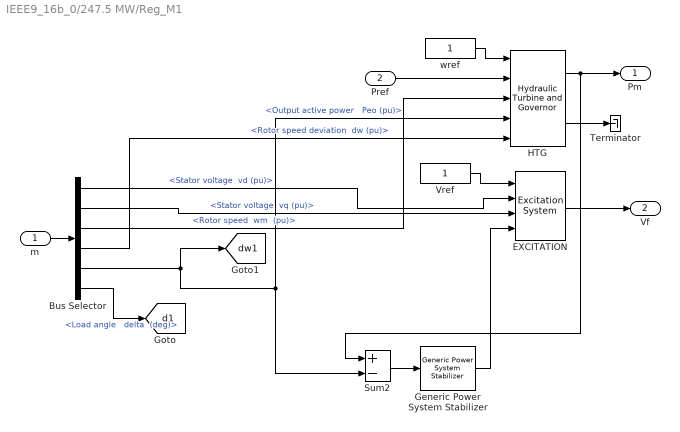
== system IEEE9_16b_0/247.5 MW/Reg_M1 ==
  m : Inport
  Pref : Inport  Port=2
  Bus Selector : BusSelector  OutputSignals="dq0 components.Stator voltage  vd (pu),dq0 components.Stator voltage  vq (pu),Mechanical.Rotor speed  wm  (pu),Mechanical.Rotor speed deviation  dw (pu),Output active power   Peo (pu),Load angle   delta  (deg)"
  EXCITATION : sps_avr/Excitation System  tr=20e-3  reg=[ 200, 0.001 ]  exc=[ 1, 0 ]  tgr=[ 0, 0 ]  damp=[ 0.001, 0.1 ]  sat=[ 0, 0 ]  lim="[ 0,  7, 0 ]"  v0=[1 1.1938]
      settings: SourceProductBaseCode=PS
  Generic Power System Stabilizer : powerlib/Machines/Generic Power System Stabilizer  Tsensor=15e-3  K=2.5  Twashout=1  Tleadlag1="[0.06  1]"  Tleadlag2="[0  0]"  VSlimits=[-0.15 0.15]  Vinit=0  Plot_On=off  MagdB_On=on  FreqRange=logspace(-2,2,500)
      settings: SourceProductBaseCode=PS
  HTG : powerlib/Machines/Hydraulic Turbine and Governor  sm="[ 10/3  0.07 ]"  gate="[  0.01  0.97518  -0.1  0.1 ]"  reg="[  0.05  1.163  0.105  0  0.01  ]"  hyd="[  0  2.67  ]"  dref=0  po=0.51299
      settings: SourceProductBaseCode=PS
  Sum2 : Sum  Inputs=+-  InputSameDT=on  SaturateOnIntegerOverflow=on  OutDataTypeStr=Inherit: Same as first input
  Terminator : Terminator
  Vref : Constant
  wref : Constant
  Pm : Outport  InitialOutput=0
  Vf : Outport  Port=2  InitialOutput=0
  tag scope: d1=global, dw1=global
  wires:
  HTG/2 -> Terminator/1
  Vref/1 -> EXCITATION/1
  m/1 -> Bus Selector/1
  Bus Selector/4 -> HTG/5  "<Rotor speed deviation  dw (pu)>"
  Bus Selector/5 -> [dw1], HTG/4, Sum2/2  "<Output active power   Peo (pu)>"
  Bus Selector/3 -> HTG/3  "<Rotor speed  wm  (pu)>"
  Pref/1 -> HTG/2
  wref/1 -> HTG/1
  HTG/1 -> Pm/1, Sum2/1
  Bus Selector/2 -> EXCITATION/3  "<Stator voltage  vq (pu)>"
  EXCITATION/1 -> Vf/1
  Bus Selector/1 -> EXCITATION/2  "<Stator voltage  vd (pu)>"
  Generic Power System Stabilizer/1 -> EXCITATION/4
  Sum2/1 -> Generic Power System Stabilizer/1
  Bus Selector/6 -> [d1]  "<Load angle   delta  (deg)>"

== matlab function IEEE9_16b_0/Relay/MATLAB Function ==
  settings: updateMethod=DISCRETE
  data: Vabc input; Za output; Iabc input; Zb output; Zc output; Zab output; Zbc output; Zca output; Za_3ph output; Zb_3ph output; Zc_3ph output; T1 output; T2 output; T3 output
function [Za, Zb, Zc, Zab, Zbc, Zca, Za_3ph, Zb_3ph, Zc_3ph, T1, T2, T3] = fcn(Vabc, Iabc)
 
persistent init C1 C2 C3 r1 r2 r3 trip1 trip2 trip3 k
if isempty(init)  
    trip1 = false; trip2 = false; trip3 = false;
    Zline = 100*(0.0449 + 1i*2*pi*60*1.01e-3);
    Z0_line = 100*(0.11241 + 1i*60*2.02e-3*2*pi);
    k = (Z0_line - Zline)./Zline;
    Z1 = 0.80*Zline;
    Z2 = 1.2*Zline;
    Z3 = 2*abs(Zline)*exp(1i*80*pi/180);
    C1 = Z1/2; C2 = Z2/2; C3 = Z3/2;
    r1 = abs(C1); r2 = abs(C2); r3 = abs(C3);
    MTA1 = angle(Z1);
    MTA2 = angle(Z2);
    MTA3 = 80*pi/180;
    init = 1;
    
%     circle(real(C1),imag(C1),r1)
%     circle(real(C2),imag(C2),r2)
%     circle(real(C3),imag(C3),r3)
end

Va = Vabc(1); Vb = Vabc(2); Vc = Vabc(3);
Ia = Iabc(1); Ib = Iabc(2); Ic =Iabc(3);
Io = (Ia+Ib+Ic)/3;

Za = Va/(Ia+k*Io);
Zb = Vb/(Ib+k*Io);
Zc = Vc/(Ic+k*Io);
Zab = (Va-Vb)/(Ia-Ib);
Zbc = (Vb-Vc)/(Ib-Ic);
Zca = (Vc-Va)/(Ic-Ia);
Za_3ph = Va/Ia;
Zb_3ph = Vb/Ib;
Zc_3ph = Vc/Ic;

if any([abs(Za-C1),abs(Zb-C1),abs(Zc-C1),abs(Zab-C1),abs(Zbc-C1),abs(Zca-C1),abs(Za_3ph-C1),abs(Zb_3ph-C1),abs(Zc_3ph-C1)] <= r1)
    trip1 = true;
elseif any([abs(Za-C2),abs(Zb-C2),abs(Zc-C2),abs(Zab-C2),abs(Zbc-C2),abs(Zca-C2),abs(Za_3ph-C2),abs(Zb_3ph-C2),abs(Zc_3ph-C2)] <= r2)
    trip2 = true;
elseif any([abs(Za-C3),abs(Zb-C3),abs(Zc-C3),abs(Zab-C3),abs(Zbc-C3),abs(Zca-C3),abs(Za_3ph-C3),abs(Zb_3ph-C3),abs(Zc_3ph-C3)] <= r3)
    trip3 = true;
end

T1 =trip1; T2 = trip2; T3 = trip3;
end
